simulink model "drawWorks_Sim_GenericDrive"  (R2017b)
settings: Solver=ode45  StartTime=0.0  StopTime=30  FixedStep=Ts  RelTol=1e-3  AbsTol=1e-3  EnableMultiTasking=on
PreLoadFcn:
  | addpath('./Images');
  | addpath('./Simscape_Pulley_Library');
InitFcn:
  | DrawworksParameters();
values from neighbouring files (symbols this model uses):
  n = 6    [DrawworksParameters.m]
  Tssc = 10*Ts    (= 0.0015)    [DrawworksParameters.m]
undefined symbols (not defined in the file or in its folder): Drum, Tackle
libraries: fl_lib x24, CustomComponents_lib x11, nesl_utility x11, sdl_lib x3, simulink x2
Description:
  | Copyright 2008-2016 The MathWorks, Inc.
settings Model: ExtModeAutoUpdateStatusClock=off  Creator=MathWorks  LastModifiedBy=jlesage
settings DataIOCC: LimitDataPoints=on  SaveFormat=Array  SignalLoggingSaveFormat=ModelDataLogs  SaveOutput=off  SignalLogging=off  SaveTime=off  SignalLoggingName=sigsOut
settings OptimizationCC: ExpressionDepthLimit=2147483647  InitFltsAndDblsToZero=on  LifeSpan=inf
settings DebuggingCC: UnderspecifiedInitializationDetection=Classic  MergeDetectMultiDrivingBlocksExec=none  CheckExecutionContextPreStartOutputMsg=on  CheckExecutionContextRuntimeOutputMsg=on  SignalResolutionControl=TryResolveAllWithWarning  MultiTaskDSMMsg=warning  MultiTaskCondExecSysMsg=none  FcnCallInpInsideContextMsg=warning  StateNameClashWarn=warning  SFUnexpectedBacktrackingDiag=warning  SFNoUnconditionalDefaultTransitionDiag=warning  SFExecutionAtInitializationDiag=none
settings HardwareCC: ProdBitPerPointer=32  ProdBitPerSizeT=32  ProdBitPerPtrDiffT=32  ProdLargestAtomicFloat=None  ProdIntDivRoundTo=Undefined  ProdEndianess=Unspecified  ProdWordSize=32  ProdHWDeviceType=32-bit Generic  TargetUnknown=on
settings ModelReferenceCC: PropagateSignalLabelsOutOfModel=off
settings CodeAppCC: StateflowObjectComments=on
settings GRTTargetCC: TargetLangStandard=C89/C90 (ANSI)  GeneratePreprocessorConditionals=Disable all  CombineOutputUpdateFcns=off  GRTInterface=on
settings ConfigComp: CovMetricSettings=dw  CovHtmlReporting=on  CovSaveCumulativeToWorkspaceVar=on  CovSaveSingleToWorkspaceVar=on  CovExternalEMLEnable=off  CovSFcnEnable=off
settings SimscapeCC: SimscapeNormalizeSystem=off

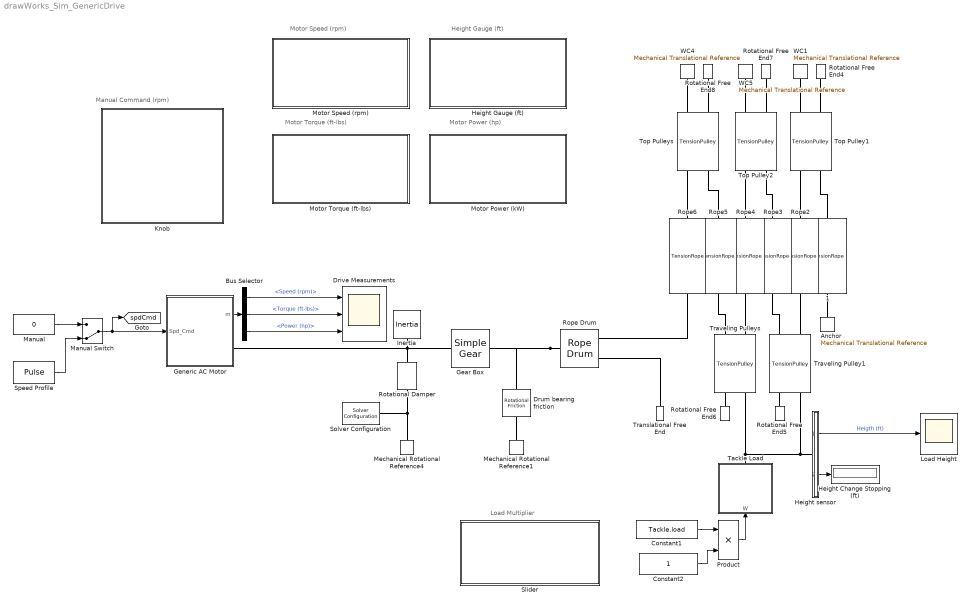
== system drawWorks_Sim_GenericDrive ==
  note: Motor Speed (rpm)
  note: Height Gauge (ft)
  note: Motor Torque (ft-lbs)
  note: Motor Power (hp)
  note: Manual Command (rpm)
  note: Load Multiplier
  1 : CustomComponents_lib/TensionRope  rope_stiff=Rope.stiffness N/m  damping=Rope.damping N/(m/s)  L0=10 m  mass=1 kg  s_specify=off  s_priority=High  s=0.08 m  s_nominal_specify=off  s_nominal_unit=m  s_nominal_value=1  L_specify=off  L_priority=High  L=1 m  L_nominal_specify=off  L_nominal_unit=m  L_nominal_value=1  f_specify=on  f_priority=High  f=Tackle.load/n N  f_nominal_specify=off  f_nominal_unit=N  f_nominal_value=1  v_specify=off  v_priority=High  v=0 m/s  v_nominal_specify=off  v_nominal_unit=m/s  v_nominal_value=1  fd_specify=off  fd_priority=High  fd=0 N  fd_nominal_specify=off  fd_nominal_unit=N  fd_nominal_value=1  fs_specify=off  fs_priority=High  fs=0 N  fs_nominal_specify=off  fs_nominal_unit=N  fs_nominal_value=1
  Anchor : fl_lib/Mechanical/Translational Elements/Mechanical Translational Reference
  Bus Selector : BusSelector  OutputSignals=Speed (rpm),Torque (ft-lbs),Power (hp)
  Constant1 : Constant  Value=Tackle.load
  Constant2 : Constant
  Drive Measurements : Scope  NumInputPorts=3
  Drum bearing friction : fl_lib/Mechanical/Rotational Elements/Rotational Friction  brkwy_trq=Drum.friction*1.1 N*m  brkwy_vel=0.060623 rad/s  Col_trq=Drum.friction N*m  visc_coef=Drum.viscous N*m/(rad/s)  w_specify=on  w_priority=Low  w=0 rad/s  w_nominal_specify=off  w_nominal_unit=rad/s  w_nominal_value=1  t_specify=off  t_priority=High  t=0 N*m  t_nominal_specify=off  t_nominal_unit=N*m  t_nominal_value=1
      settings: SourceProductName=Simscape
  Gear Box : sdl_lib/Gears/Simple Gear  ratio=10  rotation_direction=2  friction_model=1  T_noload=0.1 N*m  T_nom=5 N*m  efficiency_nom=0.8  efficiency=0.8  mu_visc=[ 0 0 ] N*m/(rad/s)  w_thr=0.01 rad/s  pwr_thr=0.001 W  temperature_TLU=[ 280 300 320 ] K  load_TLU=[ 1 5 10 ] N*m  efficiency_TLU=[ 0.95 0.9 0.85 ]  efficiency_TLU2=[ 0.85 0.8 0.75; 0.95 0.9 0.85; 0.85 0.8 0.7 ]  thermal_mass=50 J/K  T_init=300 K
      settings: SourceProductName=Simscape Driveline
  Generic AC Motor : Subsystem  mask{Tmax=8000, Pmax=1000, wmax=1500, wrate=400}
      mask prompts: Tmax "Max Torque (ft-lbs)"; Pmax "Max Power (hp)"; wmax "Max Speed (rpm)"; wrate "Speed rate (rpm/s)"
  Height sensor : Subsystem
  Height Change Stopping (ft) : Display
  Height Gauge (ft) : Subsystem  DialogController=hmiCreateDDGDialog  IsWebBlock=on  mask(MathWorksWebBlock){webBlockId=c5aa380d-2f8e-459f-9f85-e92ca37c4779, webBlockType=semicirculargauge, ShowInLibBrowser=on, ShowInitialText=on, HMISrcModelName=drawWorks_Sim_GenericDrive}
      mask prompts: webBlockId "WebBlock Id"; webBlockType "WebBlock Type"; HMISrcModelName "Source Model"
      mask Help: helpview([docroot '/mapfiles/simulink.map'], 'hmi_half_gauge')
      mask Display:
      | if strcmp(get_param(bdroot(gcb),'BlockDiagramType'), 'library')
      |     image([(matlabroot) '/toolbox/simulink/hmi/icons/SemicircularGauge.png']);
      | end
  Inertia : fl_lib/Mechanical/Rotational Elements/Inertia  inertia=0.01 kg*m^2  w_specify=off  w_priority=High  w=0 rad/s  w_nominal_specify=off  w_nominal_unit=rad/s  w_nominal_value=1  t_specify=off  t_priority=High  t=0 N*m  t_nominal_specify=off  t_nominal_unit=N*m  t_nominal_value=1
  Knob : Subsystem  DialogController=hmiCreateDDGDialog  IsWebBlock=on  mask(MWDashboardBlock){webBlockId=b3dd6734-29cc-4e38-a886-5498566ea54e, webBlockType=continuousknob, ShowInLibBrowser=on, ShowInitialText=on, HMISrcModelName=drawWorks_Sim_GenericDrive}
      mask prompts: webBlockId "WebBlock Id"; webBlockType "WebBlock Type"; HMISrcModelName "Source Model"
      mask help: SimulinkHMI:dialogs:ContinuousKnobDialogDesc
      mask Help: helpview([docroot '/mapfiles/simulink.map'], 'hmi_knob')
      mask Display:
      | if strcmp(get_param(bdroot(gcb),'BlockDiagramType'), 'library')
      |     image([(matlabroot) '/toolbox/simulink/hmi/icons/ContinuousKnob.png']);
      | end
  Load Height : Scope
  Manual : Constant  Value=0
  Manual Switch : ManualSwitch  CurrentSetting=0
  Mechanical Rotational Reference1 : fl_lib/Mechanical/Rotational Elements/Mechanical Rotational Reference
  Mechanical Rotational Reference4 : fl_lib/Mechanical/Rotational Elements/Mechanical Rotational Reference
  Motor Power (kW) : Subsystem  DialogController=hmiCreateDDGDialog  IsWebBlock=on  mask(MathWorksWebBlock){webBlockId=19b5fd22-3d9e-453c-98f3-af57f09a4a2a, webBlockType=semicirculargauge, ShowInLibBrowser=on, ShowInitialText=on, HMISrcModelName=drawWorks_Sim_GenericDrive}
      mask prompts: webBlockId "WebBlock Id"; webBlockType "WebBlock Type"; HMISrcModelName "Source Model"
      mask Help: helpview([docroot '/mapfiles/simulink.map'], 'hmi_half_gauge')
      mask Display:
      | if strcmp(get_param(bdroot(gcb),'BlockDiagramType'), 'library')
      |     image([(matlabroot) '/toolbox/simulink/hmi/icons/SemicircularGauge.png']);
      | end
  Motor Speed (rpm) : Subsystem  DialogController=hmiCreateDDGDialog  IsWebBlock=on  mask(MathWorksWebBlock){webBlockId=7eba74a7-8cbb-4d45-95db-04e3d24d85db, webBlockType=semicirculargauge, ShowInLibBrowser=on, ShowInitialText=on, HMISrcModelName=drawWorks_Sim_GenericDrive}
      mask prompts: webBlockId "WebBlock Id"; webBlockType "WebBlock Type"; HMISrcModelName "Source Model"
      mask Help: helpview([docroot '/mapfiles/simulink.map'], 'hmi_half_gauge')
      mask Display:
      | if strcmp(get_param(bdroot(gcb),'BlockDiagramType'), 'library')
      |     image([(matlabroot) '/toolbox/simulink/hmi/icons/SemicircularGauge.png']);
      | end
  Motor Torque (ft-lbs) : Subsystem  DialogController=hmiCreateDDGDialog  IsWebBlock=on  mask(MathWorksWebBlock){webBlockId=3687f525-ad22-450b-a80e-b9211f80e0d5, webBlockType=semicirculargauge, ShowInLibBrowser=on, ShowInitialText=on, HMISrcModelName=drawWorks_Sim_GenericDrive}
      mask prompts: webBlockId "WebBlock Id"; webBlockType "WebBlock Type"; HMISrcModelName "Source Model"
      mask Help: helpview([docroot '/mapfiles/simulink.map'], 'hmi_half_gauge')
      mask Display:
      | if strcmp(get_param(bdroot(gcb),'BlockDiagramType'), 'library')
      |     image([(matlabroot) '/toolbox/simulink/hmi/icons/SemicircularGauge.png']);
      | end
  Product : Product
  Rope Drum : sdl_lib/Couplings & Drives/Rope Drum  r_drum=Drum.radius m  windup=2  check_tension=1  b_drum=0 N*m/(rad/s)  model_inertia=1  inertia=Drum.inertia kg*m^2  initial_velocity=0 rad/s
      settings: SourceProductName=Simscape Driveline  SourceProductBaseCode=LD
  Rope{2..6} (5 alike) : CustomComponents_lib/TensionRope  rope_stiff=Rope.stiffness N/m  damping=Rope.damping N/(m/s)  L0=10 m  mass=1 kg  s_specify=off  s_priority=High  s=0.08 m  s_nominal_specify=off  s_nominal_unit=m  s_nominal_value=1  L_specify=off  L_priority=High  L=1 m  L_nominal_specify=off  L_nominal_unit=m  L_nominal_value=1  f_specify=on  f_priority=High  f=Tackle.load/n N  f_nominal_specify=off  f_nominal_unit=N  f_nominal_value=1  v_specify=off  v_priority=High  v=0 m/s  v_nominal_specify=off  v_nominal_unit=m/s  v_nominal_value=1  fd_specify=off  fd_priority=High  fd=0 N  fd_nominal_specify=off  fd_nominal_unit=N  fd_nominal_value=1  fs_specify=off  fs_priority=High  fs=0 N  fs_nominal_specify=off  fs_nominal_unit=N  fs_nominal_value=1
  Rotational Damper : fl_lib/Mechanical/Rotational Elements/Rotational Damper  D=0.001 N*m/(rad/s)  w_specify=off  w_priority=High  w=0 rad/s  w_nominal_specify=off  w_nominal_unit=rad/s  w_nominal_value=1  t_specify=off  t_priority=High  t=0 N*m  t_nominal_specify=off  t_nominal_unit=N*m  t_nominal_value=1
  Rotational Free End{4..8} (5 alike) : fl_lib/Mechanical/Rotational Elements/Rotational Free End  w_specify=off  w_priority=High  w=0 rad/s  w_nominal_specify=off  w_nominal_unit=rad/s  w_nominal_value=1
      settings: SourceProductName=Simscape  SourceProductBaseCode=SS
  Slider : Subsystem  DialogController=hmiCreateDDGDialog  IsWebBlock=on  mask(MWDashboardBlock){webBlockId=0993a495-73f7-4df6-a704-f2e0e4754f77, webBlockType=slider, ShowInLibBrowser=on, ShowInitialText=on, HMISrcModelName=drawWorks_Sim_GenericDrive}
      mask prompts: webBlockId "WebBlock Id"; webBlockType "WebBlock Type"; HMISrcModelName "Source Model"
      mask help: SimulinkHMI:dialogs:SliderDialogDesc
      mask Help: helpview([docroot '/mapfiles/simulink.map'], 'hmi_slider')
      mask Display:
      | if strcmp(get_param(bdroot(gcb),'BlockDiagramType'), 'library')
      |     image([(matlabroot) '/toolbox/simulink/hmi/icons/Slider.png']);
      | end
  Solver Configuration : nesl_utility/Solver Configuration  PhysicalDomain=network_engine_domain  SubClassName=solver  LeftPortType=input  RightPortType=generic  Accelerate=off  Tones=[]  Harmonics=[]  SimulateNoise=off  Profile=off  UseLocalSampling=off  EnableSwitchedLinearOptims=on  FrequencyDomain=off  UseCCode=off  RelTol=0.001  AbsTol=1e-06  MinStep=1e-09  ToWorkspace=off  RevertToSquareIcSolve=off  NumHomotopyIterations=100  PhasorMode=off  PhasorModeNumHarmonics=1  DoDC=off  ResidualTolerance=1e-09  UseLocalSolver=on  LocalSolverChoice=NE_BACKWARD_EULER_ADVANCER  LocalSolverSampleTime=Tssc  DoFixedCost=on  MaxNonlinIter=3  MaxModeIter=2  LinearAlgebra=Sparse  DelaysMemoryBudget=1024  AutomaticFiltering=on  FilteringTimeConstant=0.001
  Speed Profile : DiscretePulseGenerator  PulseType=Time based  Amplitude=750  Period=30  PulseWidth=50  PhaseDelay=2.5
  Tackle Load : Subsystem
      mask Display: image('tackle.jpg')
  Top Pulley1 : CustomComponents_lib/TensionPulley  radius=Pulley.radius m  b_damp=Pulley.viscous N*m/(rad/s)  inertia=Pulley.inertia kg*m^2  mass=1 kg  mu_s=1  f_A_specify=off  f_A_priority=High  f_A=0 N  f_A_nominal_specify=off  f_A_nominal_unit=N  f_A_nominal_value=1  f_B_specify=off  f_B_priority=High  f_B=0 N  f_B_nominal_specify=off  f_B_nominal_unit=N  f_B_nominal_value=1  f_C_specify=off  f_C_priority=High  f_C=0 N  f_C_nominal_specify=off  f_C_nominal_unit=N  f_C_nominal_value=1  tau_specify=off  tau_priority=High  tau=0 N*m  tau_nominal_specify=off  tau_nominal_unit=N*m  tau_nominal_value=1  w_specify=off  w_priority=High  w=0 rad/s  w_nominal_specify=off  w_nominal_unit=rad/s  w_nominal_value=1  v_specify=off  v_priority=High  v=0 m/s  v_nominal_specify=off  v_nominal_unit=m/s  v_nominal_value=1
  Top Pulley2 : CustomComponents_lib/TensionPulley  radius=Pulley.radius m  b_damp=Pulley.viscous N*m/(rad/s)  inertia=Pulley.inertia kg*m^2  mass=1 kg  mu_s=1  f_A_specify=off  f_A_priority=High  f_A=0 N  f_A_nominal_specify=off  f_A_nominal_unit=N  f_A_nominal_value=1  f_B_specify=off  f_B_priority=High  f_B=0 N  f_B_nominal_specify=off  f_B_nominal_unit=N  f_B_nominal_value=1  f_C_specify=off  f_C_priority=High  f_C=0 N  f_C_nominal_specify=off  f_C_nominal_unit=N  f_C_nominal_value=1  tau_specify=off  tau_priority=High  tau=0 N*m  tau_nominal_specify=off  tau_nominal_unit=N*m  tau_nominal_value=1  w_specify=off  w_priority=High  w=0 rad/s  w_nominal_specify=off  w_nominal_unit=rad/s  w_nominal_value=1  v_specify=off  v_priority=High  v=0 m/s  v_nominal_specify=off  v_nominal_unit=m/s  v_nominal_value=1
  Top Pulleys : CustomComponents_lib/TensionPulley  radius=Pulley.radius m  b_damp=Pulley.viscous N*m/(rad/s)  inertia=Pulley.inertia kg*m^2  mass=1 kg  mu_s=1  f_A_specify=off  f_A_priority=High  f_A=0 N  f_A_nominal_specify=off  f_A_nominal_unit=N  f_A_nominal_value=1  f_B_specify=off  f_B_priority=High  f_B=0 N  f_B_nominal_specify=off  f_B_nominal_unit=N  f_B_nominal_value=1  f_C_specify=off  f_C_priority=High  f_C=0 N  f_C_nominal_specify=off  f_C_nominal_unit=N  f_C_nominal_value=1  tau_specify=off  tau_priority=High  tau=0 N*m  tau_nominal_specify=off  tau_nominal_unit=N*m  tau_nominal_value=1  w_specify=off  w_priority=High  w=0 rad/s  w_nominal_specify=off  w_nominal_unit=rad/s  w_nominal_value=1  v_specify=off  v_priority=High  v=0 m/s  v_nominal_specify=off  v_nominal_unit=m/s  v_nominal_value=1
  Translational Free End : fl_lib/Mechanical/Translational Elements/Translational Free End  v_specify=off  v_priority=High  v=0 m/s  v_nominal_specify=off  v_nominal_unit=m/s  v_nominal_value=1
      settings: SourceProductName=Simscape  SourceProductBaseCode=SS
  Traveling Pulley1 : CustomComponents_lib/TensionPulley  radius=Pulley.radius m  b_damp=Pulley.viscous N*m/(rad/s)  inertia=Pulley.inertia kg*m^2  mass=1 kg  mu_s=1  f_A_specify=off  f_A_priority=High  f_A=0 N  f_A_nominal_specify=off  f_A_nominal_unit=N  f_A_nominal_value=1  f_B_specify=off  f_B_priority=High  f_B=0 N  f_B_nominal_specify=off  f_B_nominal_unit=N  f_B_nominal_value=1  f_C_specify=off  f_C_priority=High  f_C=0 N  f_C_nominal_specify=off  f_C_nominal_unit=N  f_C_nominal_value=1  tau_specify=off  tau_priority=High  tau=0 N*m  tau_nominal_specify=off  tau_nominal_unit=N*m  tau_nominal_value=1  w_specify=off  w_priority=High  w=0 rad/s  w_nominal_specify=off  w_nominal_unit=rad/s  w_nominal_value=1  v_specify=off  v_priority=High  v=0 m/s  v_nominal_specify=off  v_nominal_unit=m/s  v_nominal_value=1
  Traveling Pulleys : CustomComponents_lib/TensionPulley  radius=Pulley.radius m  b_damp=Pulley.viscous N*m/(rad/s)  inertia=Pulley.inertia kg*m^2  mass=1 kg  mu_s=1  f_A_specify=off  f_A_priority=High  f_A=0 N  f_A_nominal_specify=off  f_A_nominal_unit=N  f_A_nominal_value=1  f_B_specify=off  f_B_priority=High  f_B=0 N  f_B_nominal_specify=off  f_B_nominal_unit=N  f_B_nominal_value=1  f_C_specify=off  f_C_priority=High  f_C=0 N  f_C_nominal_specify=off  f_C_nominal_unit=N  f_C_nominal_value=1  tau_specify=off  tau_priority=High  tau=0 N*m  tau_nominal_specify=off  tau_nominal_unit=N*m  tau_nominal_value=1  w_specify=off  w_priority=High  w=0 rad/s  w_nominal_specify=off  w_nominal_unit=rad/s  w_nominal_value=1  v_specify=off  v_priority=High  v=0 m/s  v_nominal_specify=off  v_nominal_unit=m/s  v_nominal_value=1
  WC1 : fl_lib/Mechanical/Translational Elements/Mechanical Translational Reference
  WC4 : fl_lib/Mechanical/Translational Elements/Mechanical Translational Reference
  WC5 : fl_lib/Mechanical/Translational Elements/Mechanical Translational Reference
  tag scope: spdCmd=global
  wires:
  Generic AC Motor/1(m) -> Bus Selector/1
  Height sensor/1(x) -> Load Height/1  "Heigth (ft)"
  Manual/1 -> Manual Switch/1
  Manual Switch/1 -> Generic AC Motor/1(Spd_Cmd), [spdCmd]
  Speed Profile/1 -> Manual Switch/2
  Height sensor/2(h) -> Height Change Stopping (ft)/1
  Bus Selector/2 -> Drive Measurements/2  "<Torque (ft-lbs)>"
  Bus Selector/1 -> Drive Measurements/1  "<Speed (rpm)>"
  Bus Selector/3 -> Drive Measurements/3  "<Power (hp)>"
  Constant1/1 -> Product/1
  Constant2/1 -> Product/2
  Product/1 -> Tackle Load/1(W)
  connections:
  Tackle Load/RConn1 -- Traveling Pulleys/LConn1 -- Traveling Pulley1/LConn1 -- Height sensor/LConn1
  Rope Drum/LConn1 -- Drum bearing friction/LConn1 -- Gear Box/RConn1
  Inertia/LConn1 -- Generic AC Motor/RConn1 -- Gear Box/LConn1 -- Rotational Damper/LConn1
  Rope5/RConn1 -- Top Pulleys/RConn2
  WC1/LConn1 -- Top Pulley1/LConn1
  Rope6/RConn1 -- Top Pulleys/RConn1
  Anchor/LConn1 -- 1/LConn1
  Top Pulley2/RConn2 -- Rope3/RConn1
  Rope5/LConn1 -- Traveling Pulleys/RConn2
  WC5/LConn1 -- Top Pulley2/LConn1
  Rope Drum/RConn1 -- Translational Free End/LConn1
  Rotational Free End6/LConn1 -- Traveling Pulleys/LConn2
  Rope4/LConn1 -- Traveling Pulleys/RConn1
  Rope Drum/RConn2 -- Rope6/LConn1
  Rotational Free End4/LConn1 -- Top Pulley1/LConn2
  Rotational Damper/RConn1 -- Mechanical Rotational Reference4/LConn1 -- Solver Configuration/RConn1
  Rope4/RConn1 -- Top Pulley2/RConn1
  Rope2/RConn1 -- Top Pulley1/RConn1
  WC4/LConn1 -- Top Pulleys/LConn1
  Drum bearing friction/RConn1 -- Mechanical Rotational Reference1/LConn1
  1/RConn1 -- Top Pulley1/RConn2
  Rotational Free End5/LConn1 -- Traveling Pulley1/LConn2
  Rotational Free End7/LConn1 -- Top Pulley2/LConn2
  Rope3/LConn1 -- Traveling Pulley1/RConn2
  Rotational Free End8/LConn1 -- Top Pulleys/LConn2
  Rope2/LConn1 -- Traveling Pulley1/RConn1

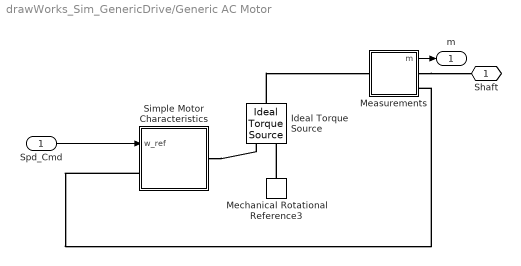
== system drawWorks_Sim_GenericDrive/Generic AC Motor ==
  Spd_Cmd : Inport
  Ideal Torque Source : fl_lib/Mechanical/Mechanical Sources/Ideal Torque Source
  Measurements : Subsystem
  Mechanical Rotational Reference3 : fl_lib/Mechanical/Rotational Elements/Mechanical Rotational Reference
  Simple Motor Characteristics : Subsystem
  Shaft : PMIOPort  Port=1  Side=Right
  m : Outport
  wires:
  Spd_Cmd/1 -> Simple Motor Characteristics/1(w_ref)
  Measurements/1(m) -> m/1
  connections:
  Measurements/RConn1 -- Shaft/RConn1
  Simple Motor Characteristics/LConn1 -- Measurements/RConn2
  Ideal Torque Source/LConn1 -- Measurements/LConn1
  Simple Motor Characteristics/RConn1 -- Ideal Torque Source/RConn1
  Mechanical Rotational Reference3/LConn1 -- Ideal Torque Source/RConn2

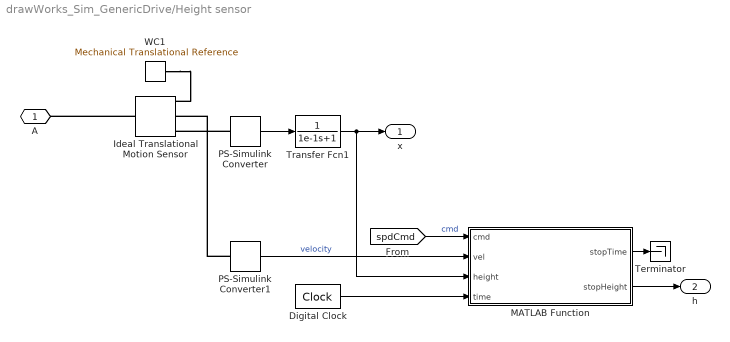
== system drawWorks_Sim_GenericDrive/Height sensor ==
  Digital Clock : DigitalClock  SampleTime=Tssc
  Ideal Translational Motion Sensor : fl_lib/Mechanical/Mechanical Sensors/Ideal Translational Motion Sensor  offset=0 m
  MATLAB Function : MATLAB Function  TreatAsAtomicUnit=on  SystemSampleTime=Tssc
  PS-Simulink Converter : nesl_utility/PS-Simulink Converter  PhysicalDomain=network_engine_domain  SubClassName=ps_output  LeftPortType=input  RightPortType=output  PseudoPeriodic=off  Frequencies=[]  Unit=ft  AffineConversion=off
  PS-Simulink Converter1 : nesl_utility/PS-Simulink Converter  PhysicalDomain=network_engine_domain  SubClassName=ps_output  LeftPortType=input  RightPortType=output  PseudoPeriodic=off  Frequencies=[]  Unit=ft/s  AffineConversion=off
  Terminator : Terminator
  Transfer Fcn1 : TransferFcn  Denominator=[1e-1 1]
  WC1 : fl_lib/Mechanical/Translational Elements/Mechanical Translational Reference
  A : PMIOPort  Port=1  Side=Left
  x : Outport
  h : Outport  Port=2
  wires:
  PS-Simulink Converter/1 -> Transfer Fcn1/1
  Transfer Fcn1/1 -> MATLAB Function/3(height), x/1
  PS-Simulink Converter1/1 -> MATLAB Function/2(vel)  "velocity"
  [spdCmd] -> MATLAB Function/1(cmd)  "cmd"
  Digital Clock/1 -> MATLAB Function/4(time)
  MATLAB Function/2(stopHeight) -> h/1
  MATLAB Function/1(stopTime) -> Terminator/1
  connections:
  PS-Simulink Converter/LConn1 -- Ideal Translational Motion Sensor/RConn3
  Ideal Translational Motion Sensor/LConn1 -- A/RConn1
  WC1/LConn1 -- Ideal Translational Motion Sensor/RConn1
  PS-Simulink Converter1/LConn1 -- Ideal Translational Motion Sensor/RConn2

== system drawWorks_Sim_GenericDrive/Height Gauge (ft) ==

== system drawWorks_Sim_GenericDrive/Knob ==

== system drawWorks_Sim_GenericDrive/Motor Power (kW) ==

== system drawWorks_Sim_GenericDrive/Motor Speed (rpm) ==

== system drawWorks_Sim_GenericDrive/Motor Torque (ft-lbs) ==

== system drawWorks_Sim_GenericDrive/Slider ==

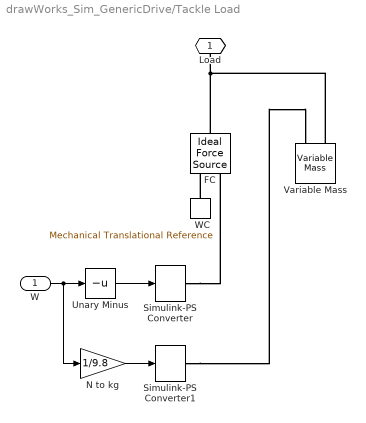
== system drawWorks_Sim_GenericDrive/Tackle Load ==
  W : Inport
  FC : fl_lib/Mechanical/Mechanical Sources/Ideal Force Source
  N to kg : Gain  Gain=1/9.8
  Simulink-PS Converter : nesl_utility/Simulink-PS Converter  PhysicalDomain=network_engine_domain  SubClassName=ps_input  LeftPortType=input  RightPortType=output  PseudoPeriodic=off  Frequencies=[]  NoiseDistribution=none  NoiseParameters=[]  Unit=N  AffineConversion=off  FilteringAndDerivatives=zero  SimscapeFilterOrder=2  InputFilterTimeConstant=0.001  UdotUserProvided=1
  Simulink-PS Converter1 : nesl_utility/Simulink-PS Converter  PhysicalDomain=network_engine_domain  SubClassName=ps_input  LeftPortType=input  RightPortType=output  PseudoPeriodic=off  Frequencies=[]  NoiseDistribution=none  NoiseParameters=[]  Unit=kg  AffineConversion=off  FilteringAndDerivatives=zero  SimscapeFilterOrder=2  InputFilterTimeConstant=0.001  UdotUserProvided=1
  Unary Minus : UnaryMinus
  Variable Mass : sdl_lib/Inertias & Loads/Variable Mass  minimum_mass=0.1 kg  p_specify=on  p_priority=High  p=0 m*kg/s  p_nominal_specify=off  p_nominal_unit=m*kg/s  p_nominal_value=1
      settings: SourceProductName=Simscape Driveline  SourceProductBaseCode=LD
  WC : fl_lib/Mechanical/Translational Elements/Mechanical Translational Reference
  Load : PMIOPort  Port=1  Side=Right
  wires:
  W/1 -> Unary Minus/1, N to kg/1
  Unary Minus/1 -> Simulink-PS Converter/1
  N to kg/1 -> Simulink-PS Converter1/1
  connections:
  WC/LConn1 -- FC/RConn2
  Simulink-PS Converter/RConn1 -- FC/RConn1
  FC/LConn1 -- Variable Mass/LConn2 -- Load/RConn1
  Simulink-PS Converter1/RConn1 -- Variable Mass/LConn1

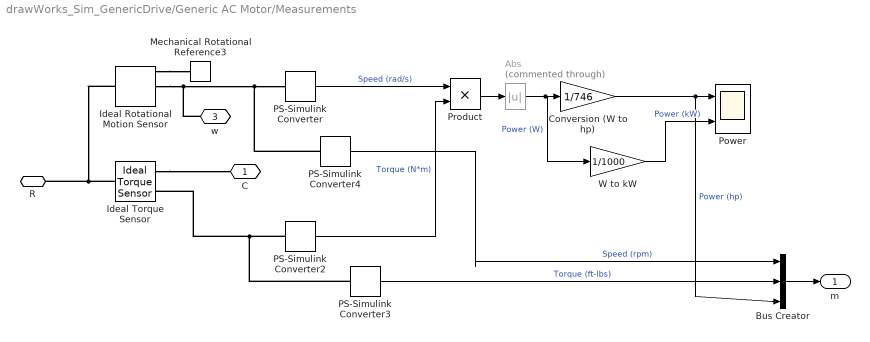
== system drawWorks_Sim_GenericDrive/Generic AC Motor/Measurements ==
  Abs : Abs  Commented=through  ZeroCross=off
  Bus Creator : BusCreator  Inputs=3
  Conversion (W to hp) : Gain  Gain=1/746
  Ideal Rotational Motion Sensor : fl_lib/Mechanical/Mechanical Sensors/Ideal Rotational Motion Sensor  offset=0 rad
  Ideal Torque Sensor : fl_lib/Mechanical/Mechanical Sensors/Ideal Torque Sensor
  Mechanical Rotational Reference3 : fl_lib/Mechanical/Rotational Elements/Mechanical Rotational Reference
  PS-Simulink Converter : nesl_utility/PS-Simulink Converter  PhysicalDomain=network_engine_domain  SubClassName=ps_output  LeftPortType=input  RightPortType=output  PseudoPeriodic=off  Frequencies=[]  Unit=rad/s  AffineConversion=off
  PS-Simulink Converter2 : nesl_utility/PS-Simulink Converter  PhysicalDomain=network_engine_domain  SubClassName=ps_output  LeftPortType=input  RightPortType=output  PseudoPeriodic=off  Frequencies=[]  Unit=N*m  AffineConversion=off
  PS-Simulink Converter3 : nesl_utility/PS-Simulink Converter  PhysicalDomain=network_engine_domain  SubClassName=ps_output  LeftPortType=input  RightPortType=output  PseudoPeriodic=off  Frequencies=[]  Unit=lbf*ft  AffineConversion=off
  PS-Simulink Converter4 : nesl_utility/PS-Simulink Converter  PhysicalDomain=network_engine_domain  SubClassName=ps_output  LeftPortType=input  RightPortType=output  PseudoPeriodic=off  Frequencies=[]  Unit=rpm  AffineConversion=off
  Power : Scope  NumInputPorts=2
  Product : Product
  W to kW : Gain  Gain=1/1000
  C : PMIOPort  Port=1  Side=Right
  R : PMIOPort  Port=2  Side=Left
  w : PMIOPort  Port=3  Side=Right
  m : Outport
  wires:
  PS-Simulink Converter/1 -> Product/1  "Speed (rad/s)"
  PS-Simulink Converter2/1 -> Product/2  "Torque (N*m)"
  Product/1 -> Abs/1
  Conversion (W to hp)/1 -> Bus Creator/3, Power/1  "Power (hp)"
  Abs/1 -> W to kW/1, Conversion (W to hp)/1  "Power (W)"
  PS-Simulink Converter3/1 -> Bus Creator/2  "Torque (ft-lbs)"
  PS-Simulink Converter4/1 -> Bus Creator/1  "Speed (rpm)"
  W to kW/1 -> Power/2  "Power (kW)"
  Bus Creator/1 -> m/1
  connections:
  Ideal Rotational Motion Sensor/RConn1 -- Mechanical Rotational Reference3/LConn1
  Ideal Torque Sensor/LConn1 -- R/RConn1 -- Ideal Rotational Motion Sensor/LConn1
  PS-Simulink Converter2/LConn1 -- PS-Simulink Converter3/LConn1 -- Ideal Torque Sensor/RConn2
  Ideal Rotational Motion Sensor/RConn2 -- w/RConn1 -- PS-Simulink Converter4/LConn1 -- PS-Simulink Converter/LConn1
  Ideal Torque Sensor/RConn1 -- C/RConn1

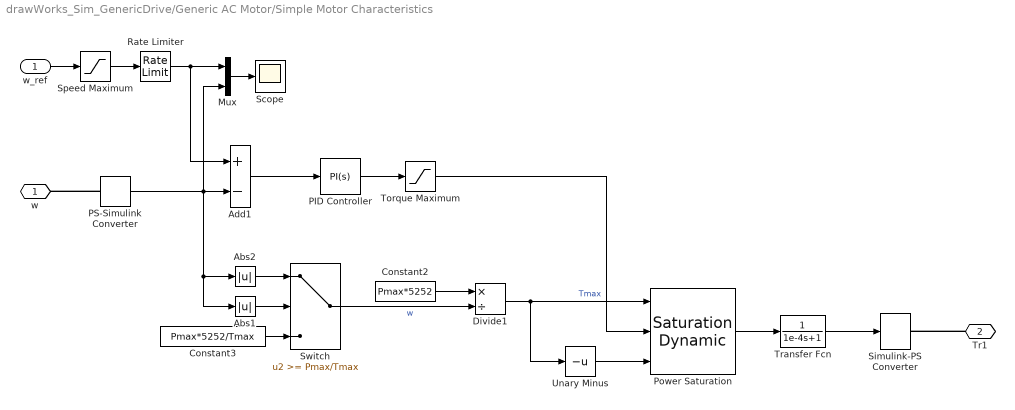
== system drawWorks_Sim_GenericDrive/Generic AC Motor/Simple Motor Characteristics ==
  w_ref : Inport
  Abs1 : Abs
  Abs2 : Abs
  Add1 : Sum  Inputs=+-
  Constant2 : Constant  Value=Pmax*5252
  Constant3 : Constant  Value=Pmax*5252/Tmax
  Divide1 : Product  Inputs=*/
  Mux : Mux  Inputs=2
  PID Controller : simulink/Continuous/PID Controller  Controller=PI  TimeDomain=Continuous-time  SampleTime=-1  IntegratorMethod=Forward Euler  FilterMethod=Forward Euler  Form=Parallel  UseFilter=on  ControllerParametersSource=internal  P=110  I=10  D=-9.19425038888835  N=3.08252405545653  InitialConditionSource=internal  InitialConditionForIntegrator=0  InitialConditionForFilter=0  ExternalReset=none  ZeroCross=off  LimitOutput=on  UpperSaturationLimit=Tmax  LowerSaturationLimit=-Tmax  LinearizeAsGain=on  AntiWindupMode=clamping  Kb=1000  TrackingMode=off  Kt=1  PParamMin=[]  PParamMax=[]  IParamMin=[]  IParamMax=[]  DParamMin=[]  DParamMax=[]  NParamMin=[]  NParamMax=[]  KbParamMin=[]  KbParamMax=[]  KtParamMin=[]  KtParamMax=[]  POutMin=[]  POutMax=[]  IOutMin=[]  IOutMax=[]  DOutMin=[]  DOutMax=[]  NOutMin=[]  NOutMax=[]  KbOutMin=[]  KbOutMax=[]  KtOutMin=[]  KtOutMax=[]  IntegratorOutMin=[]  IntegratorOutMax=[]  FilterOutMin=[]  FilterOutMax=[]  SumOutMin=[]  SumOutMax=[]  SumI1OutMin=[]  SumI1OutMax=[]  SumI2OutMin=[]  SumI2OutMax=[]  SumI3OutMin=[]  SumI3OutMax=[]  SumDOutMin=[]  SumDOutMax=[]  SaturationOutMin=[]  SaturationOutMax=[]  IntegratorContinuousStateAttributes=''  IntegratorStateMustResolveToSignalObject=off  IntegratorRTWStateStorageClass=Auto  FilterContinuousStateAttributes=''  FilterStateMustResolveToSignalObject=off  FilterRTWStateStorageClass=Auto  DifferentiatorICPrevScaledInput=0  DifferentiatorOutMin=[]  DifferentiatorOutMax=[]  InitialConditionSetting=State (most efficient)  FilterDiffOutCoefMin=[]  FilterDiffOutCoefMax=[]  SumDenOutMin=[]  SumDenOutMax=[]  SumNumOutMin=[]  SumNumOutMax=[]  ReciprocalOutMin=[]  ReciprocalOutMax=[]  DivideOutMin=[]  DivideOutMax=[]  TunerSelectOption=Transfer Function Based (PID Tuner App)
  PS-Simulink Converter : nesl_utility/PS-Simulink Converter  PhysicalDomain=network_engine_domain  SubClassName=ps_output  LeftPortType=input  RightPortType=output  PseudoPeriodic=off  Frequencies=[]  Unit=rpm  AffineConversion=off
  Power Saturation : simulink/Discontinuities/Saturation Dynamic  OutMin=[]  OutMax=[]  OutDataTypeStr=Inherit: Same as second input  OutDataType=fixdt(1, 16)  OutScaling=2^-10  DoSatur=off
  Rate Limiter : RateLimiter  RisingSlewLimit=wrate  FallingSlewLimit=-wrate  SampleTimeMode=inherited
  Scope : Scope
  Simulink-PS Converter : nesl_utility/Simulink-PS Converter  PhysicalDomain=network_engine_domain  SubClassName=ps_input  LeftPortType=input  RightPortType=output  PseudoPeriodic=off  Frequencies=[]  NoiseDistribution=none  NoiseParameters=[]  Unit=ft*lb  AffineConversion=off  FilteringAndDerivatives=filter  SimscapeFilterOrder=2  InputFilterTimeConstant=0.001  UdotUserProvided=1
  Speed Maximum : Saturate  UpperLimit=wmax  LowerLimit=-wmax  ZeroCross=off
  Switch : Switch  Threshold=Pmax/Tmax  ZeroCross=off
  Torque Maximum : Saturate  UpperLimit=Tmax  LowerLimit=-Tmax  ZeroCross=off
  Transfer Fcn : TransferFcn  Denominator=[1e-4 1]
  Unary Minus : UnaryMinus
  w : PMIOPort  Port=1  Side=Left
  Tr1 : PMIOPort  Port=2  Side=Right
  wires:
  Transfer Fcn/1 -> Simulink-PS Converter/1
  Mux/1 -> Scope/1
  Rate Limiter/1 -> Add1/1, Mux/1
  w_ref/1 -> Speed Maximum/1
  Add1/1 -> PID Controller/1
  PID Controller/1 -> Torque Maximum/1
  Torque Maximum/1 -> Power Saturation/2
  Speed Maximum/1 -> Rate Limiter/1
  PS-Simulink Converter/1 -> Abs2/1, Abs1/1, Add1/2, Mux/2
  Constant3/1 -> Switch/3
  Switch/1 -> Divide1/2  "w"
  Abs1/1 -> Switch/2
  Constant2/1 -> Divide1/1
  Divide1/1 -> Unary Minus/1, Power Saturation/1  "Tmax"
  Unary Minus/1 -> Power Saturation/3
  Abs2/1 -> Switch/1
  Power Saturation/1 -> Transfer Fcn/1
  connections:
  Tr1/RConn1 -- Simulink-PS Converter/RConn1
  PS-Simulink Converter/LConn1 -- w/RConn1

== matlab function drawWorks_Sim_GenericDrive/Height sensor/MATLAB Function ==
  data: cmd input; stopTime output; vel input; height input; time input; stopHeight output
function [stopTime,stopHeight] = fcn(cmd,vel,height,time)

persistent timeElapse
persistent measTime
persistent timeStart
persistent prevCmd
persistent heightElapse
persistent heightStart

if isempty(timeElapse) || time < 1
    timeElapse = 0;
    measTime = 0;
    timeStart = time;
    prevCmd = 0;
    heightElapse = 0;
    heightStart = 0;
else  
    if cmd == 0 && abs(cmd-prevCmd) > 1e-1 && measTime == 0
        timeStart = time;
        heightStart = height;
        measTime = 1;
    end
    
    if measTime == 1 && abs(vel) < 1e-1
        timeElapse = time - timeStart;
        heightElapse = height - heightStart;
        measTime = 0;
    end
    
    % Update each step;
    prevCmd = cmd;
    
end

stopTime = timeElapse;
stopHeight = heightElapse;
